simulink model "QuaterCar_Model"  (R2018b)
settings: Solver=VariableStepAuto  StartTime=0.0  StopTime=10.0  RelTol=1e-3
values from neighbouring files (symbols this model uses):
  cs = 1000    [SetCoefficients.m]
  g = 9.81    [SetCoefficients_QC.m]
  ks = 2e4    (= 20000)    [SetCoefficients.m]    (also in SetCoefficients_QC.m)
  kt = 14e4    (= 140000)    [SetCoefficients.m]    (also in SetCoefficients_QC.m)
  m1 = 250    [SetCoefficients.m]    (also in SetCoefficients_QC.m)
settings Model: Creator=joebe  LastModifiedBy=joebe

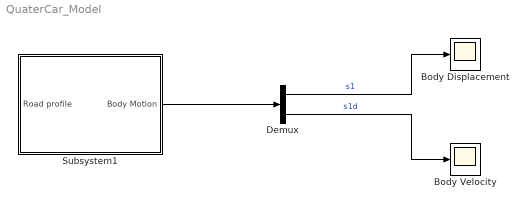
== system QuaterCar_Model ==
  Body Displacement : Scope
  Body Velocity : Scope
  Demux : Demux  Outputs=2
  Subsystem1 : Subsystem
  wires:
  Demux/1 -> Body Displacement/1  "s1"
  Demux/2 -> Body Velocity/1  "s1d"
  Subsystem1/1(Body Motion) -> Demux/1

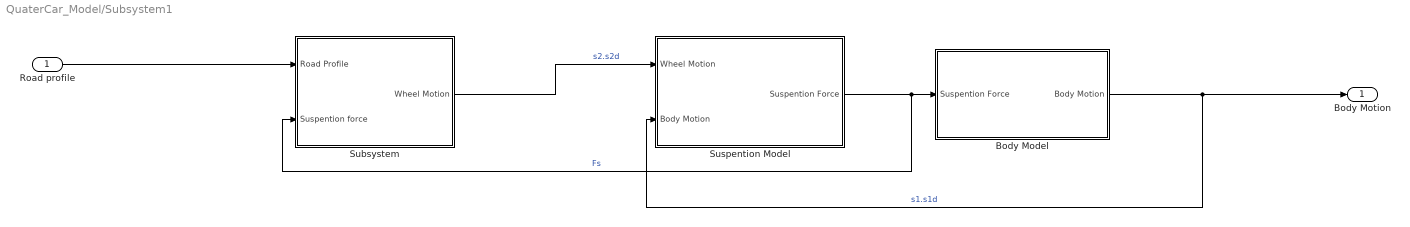
== system QuaterCar_Model/Subsystem1 ==
  Road profile : Inport
  Body Model : Subsystem
  Subsystem : Subsystem
  Suspention Model : Subsystem
  Body Motion : Outport
  wires:
  Suspention Model/1(Suspention Force) -> Subsystem/2(Suspention force), Body Model/1("Suspention Force ")  "Fs"
  Subsystem/1(Wheel Motion) -> Suspention Model/1(Wheel Motion)  "s2.s2d"
  Body Model/1(Body Motion) -> Body Motion/1, Suspention Model/2(Body Motion)  "s1.s1d"
  Road profile/1 -> Subsystem/1(Road Profile)

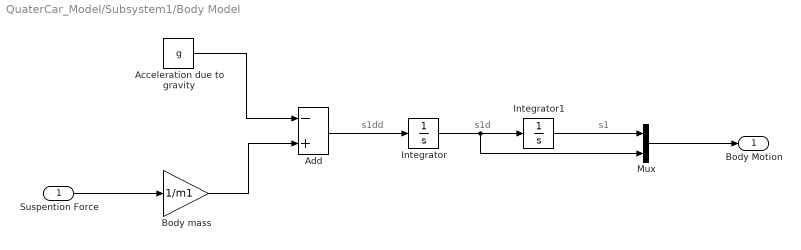
== system QuaterCar_Model/Subsystem1/Body Model ==
  note: s1d
  note: s1
  note: s1dd
  "Suspention Force " : Inport
  Acceleration due to gravity : Constant  Value=g
  Add : Sum  Inputs=-+
  Body mass : Gain  Gain=1/m1
  Integrator : Integrator
  Integrator1 : Integrator
  Mux : Mux  Inputs=2
  Body Motion : Outport
  wires:
  Body mass/1 -> Add/2
  Integrator/1 -> Mux/2, Integrator1/1
  Add/1 -> Integrator/1
  Acceleration due to gravity/1 -> Add/1
  Integrator1/1 -> Mux/1
  "Suspention Force "/1 -> Body mass/1
  Mux/1 -> Body Motion/1

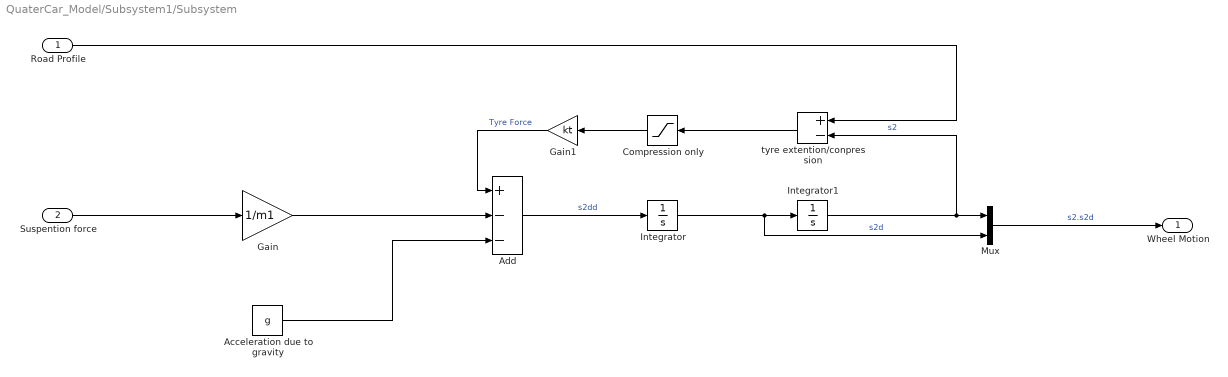
== system QuaterCar_Model/Subsystem1/Subsystem ==
  Road Profile : Inport
  Suspention force : Inport  Port=2
  Acceleration due to gravity : Constant  Value=g
  Add : Sum  Inputs=+--
  Compression only : Saturate  UpperLimit=1000  LowerLimit=0  OutMin=0  RndMeth=Nearest
  Gain : Gain  Gain=1/m1
  Gain1 : Gain  Gain=kt
  Integrator : Integrator
  Integrator1 : Integrator
  Mux : Mux  Inputs=2
  tyre extention/conpression : Sum  Inputs=+-
  Wheel Motion : Outport
  wires:
  Compression only/1 -> Gain1/1
  Integrator1/1 -> tyre extention/conpression/2, Mux/1  "s2"
  Integrator/1 -> Mux/2, Integrator1/1  "s2d"
  Add/1 -> Integrator/1  "s2dd"
  Acceleration due to gravity/1 -> Add/3
  tyre extention/conpression/1 -> Compression only/1
  Gain/1 -> Add/2
  Gain1/1 -> Add/1  "Tyre Force"
  Road Profile/1 -> tyre extention/conpression/1
  Mux/1 -> Wheel Motion/1  "s2.s2d"
  Suspention force/1 -> Gain/1

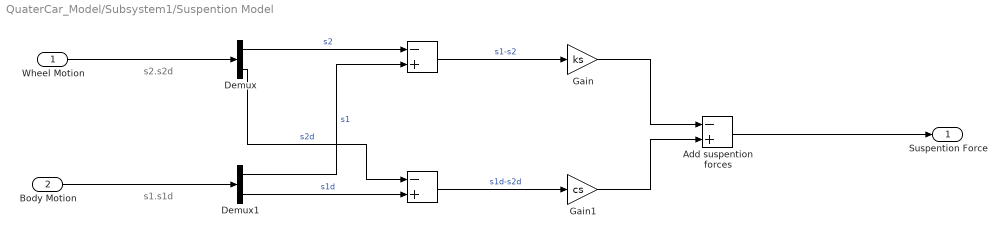
== system QuaterCar_Model/Subsystem1/Suspention Model ==
  note: s1.s1d
  note: s2.s2d
  Wheel Motion : Inport
  Body Motion : Inport  Port=2
  " " : Sum  Inputs=-+
  " " : Sum  Inputs=-+
  Add suspention forces : Sum  Inputs=-+
  Demux : Demux  Outputs=2
  Demux1 : Demux  Outputs=2
  Gain : Gain  Gain=ks
  Gain1 : Gain  Gain=cs
  Suspention Force : Outport
  wires:
  Demux1/2 -> " "/2  "s1d"
  " "/1 -> Gain/1  "s1-s2"
  Demux1/1 -> " "/2  "s1"
  Gain1/1 -> Add suspention forces/2
  Gain/1 -> Add suspention forces/1
  Demux/1 -> " "/1  "s2"
  Demux/2 -> " "/1  "s2d"
  Body Motion/1 -> Demux1/1
  " "/1 -> Gain1/1  "s1d-s2d"
  Add suspention forces/1 -> Suspention Force/1
  Wheel Motion/1 -> Demux/1
